simulink model "static_dy"  (R2020b)
settings: Solver=VariableStepAuto  StartTime=0.0  StopTime=10.0  RelTol=1e-3
values from neighbouring files (symbols this model uses):
  dqi = [0 0 0]'    [main_3DoF_robots.m]
  he = [fex fey fez uex uey uez]'    [MyRobot.m]    (also in getBHat.m = zeros(6,1); main_3DoF_robots.m = [0 0 0 0 0 0]')
  myRobot = MyRobot('PRP.urdf', DH, links)    [main_3DoF_robots.m]
  qi = [0 0 0]'    [main_3DoF_robots.m]
settings Model: Creator=simon  LastModifiedBy=simon

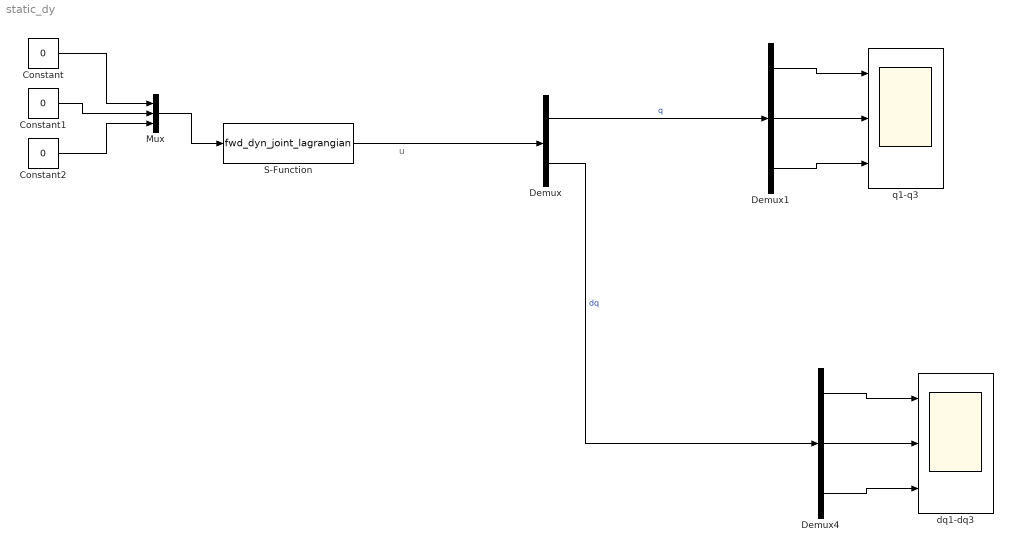
== system static_dy ==
  note: u
  Constant : Constant  Value=0
  Constant1 : Constant  Value=0
  Constant2 : Constant  Value=0
  Demux : Demux  Outputs=2
  Demux1 : Demux  Outputs=myRobot.N
  Demux4 : Demux  Outputs=myRobot.N
  Mux : Mux  Inputs=3
  S-Function : S-Function  FunctionName=fwd_dyn_joint_lagrangian  Parameters=myRobot,he,qi,dqi  SFunctionDeploymentMode=off  EnableBusSupport=off
  dq1-dq3 : Scope  NumInputPorts=3
  q1-q3 : Scope  NumInputPorts=3
  wires:
  Demux4/2 -> dq1-dq3/2
  Demux4/1 -> dq1-dq3/1
  Demux/2 -> Demux4/1  "dq"
  S-Function/1 -> Demux/1
  Demux1/3 -> q1-q3/3
  Demux1/2 -> q1-q3/2
  Demux1/1 -> q1-q3/1
  Demux/1 -> Demux1/1  "q"
  Demux4/3 -> dq1-dq3/3
  Constant/1 -> Mux/1
  Constant1/1 -> Mux/2
  Constant2/1 -> Mux/3
  Mux/1 -> S-Function/1
